simulink model "SetPoint"  (R2023a)
settings: Solver=VariableStepAuto  StartTime=0.0  StopTime=0.2  RelTol=1e-3
values from neighbouring files (symbols this model uses):
  decoupling_active = true    [PMSM.m]
  I_max = 20    [PMSM.m]
  K_Id = R_s/(2*tau_sigma)    (= 675)    [PMSM.m]
  K_Iq = R_s/(2*tau_sigma)    (= 675)    [PMSM.m]
  K_Pd = L_d/(2*tau_sigma)    (= 1.125)    [PMSM.m]
  K_Pq = L_q/(2*tau_sigma)    (= 4.5)    [PMSM.m]
  L_d = 0.00045    [PMSM.m]
  L_q = 0.0018    [PMSM.m]
  motor_type = 1    [PMSM.m]
  p = 4    [PMSM.m]
  Psi_PM = 0.0195    [PMSM.m]
  R_s = 0.27    [PMSM.m]
  Ts = 1 / PWM_frequency    (= 0.0001)    [PMSM.m]
  V_max = V_DC/sqrt(3)    [PMSM.m]
libraries: slpidlib x2
settings Model: PacingRate=0.010000  Creator=brogh  LastModifiedBy=hufnagelde
settings DataIOCC: SaveFormat=StructureWithTime
settings OptimizationCC: ReuseModelBlockBuffer=off
settings DebuggingCC: UnconnectedInputMsg=warning  UnconnectedOutputMsg=warning  UnconnectedLineMsg=warning
settings ModelReferenceCC: EnableRefExpFcnMdlSchedulingChecks=on
settings RTWCC: DLArmComputeVersion=19.05

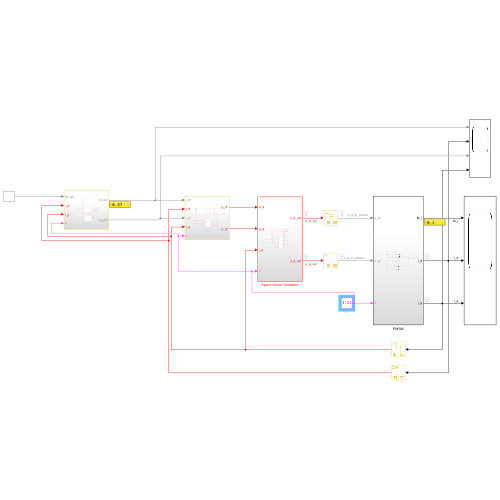
[thumbnail: Simulink's stored preview of the top-level diagram]
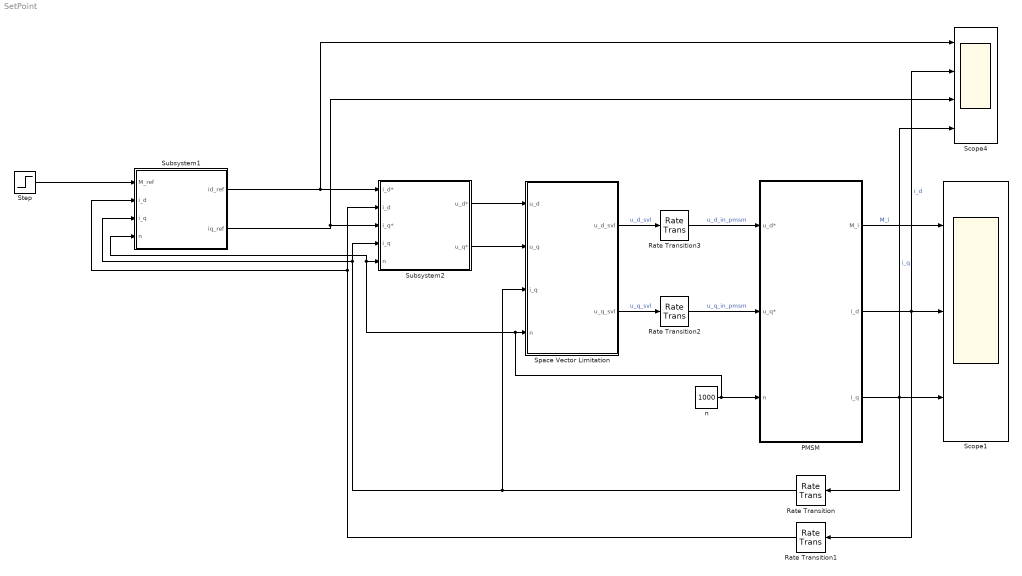
== system SetPoint ==
  PMSM : Subsystem
  Rate Transition : RateTransition  OutPortSampleTime=Ts
  Rate Transition1 : RateTransition  OutPortSampleTime=Ts
  Rate Transition2 : RateTransition  OutPortSampleTime=0
  Rate Transition3 : RateTransition  OutPortSampleTime=0
  Scope1 : Scope  NumInputPorts=3
  Scope4 : Scope  NumInputPorts=4
  Space Vector Limitation : Subsystem
  Step : Step  Time=0.03  After=0.1  SampleTime=0
  Subsystem1 : Subsystem
  Subsystem2 : Subsystem
  n : Constant  Value=1000
  wires:
  PMSM/1(M_i) -> Scope1/1  "M_i"
  PMSM/3(i_q) -> Scope4/4, Scope1/3, Rate Transition/1  "i_q"
  PMSM/2(i_d) -> Scope4/2, Scope1/2, Rate Transition1/1  "i_d"
  Rate Transition/1 -> Subsystem1/3(i_q), Subsystem2/4(i_q), Space Vector Limitation/3(i_q)
  Rate Transition2/1 -> PMSM/2(u_q*)  "u_q_in_pmsm"
  Rate Transition3/1 -> PMSM/1(u_d*)  "u_d_in_pmsm"
  Space Vector Limitation/1(u_d_svl) -> Rate Transition3/1  "u_d_svl"
  Space Vector Limitation/2(u_q_svl) -> Rate Transition2/1  "u_q_svl"
  Subsystem1/1(id_ref) -> Scope4/1, Subsystem2/1(i_d*)
  Subsystem1/2(iq_ref) -> Scope4/3, Subsystem2/3(i_q*)
  Rate Transition1/1 -> Subsystem2/2(i_d), Subsystem1/2(i_d)
  Subsystem2/1(u_d*) -> Space Vector Limitation/1(u_d)
  Subsystem2/2(u_q*) -> Space Vector Limitation/2(u_q)
  Step/1 -> Subsystem1/1(M_ref)
  n/1 -> Subsystem1/4(n), Subsystem2/5(n), Space Vector Limitation/4(n), PMSM/3(n)

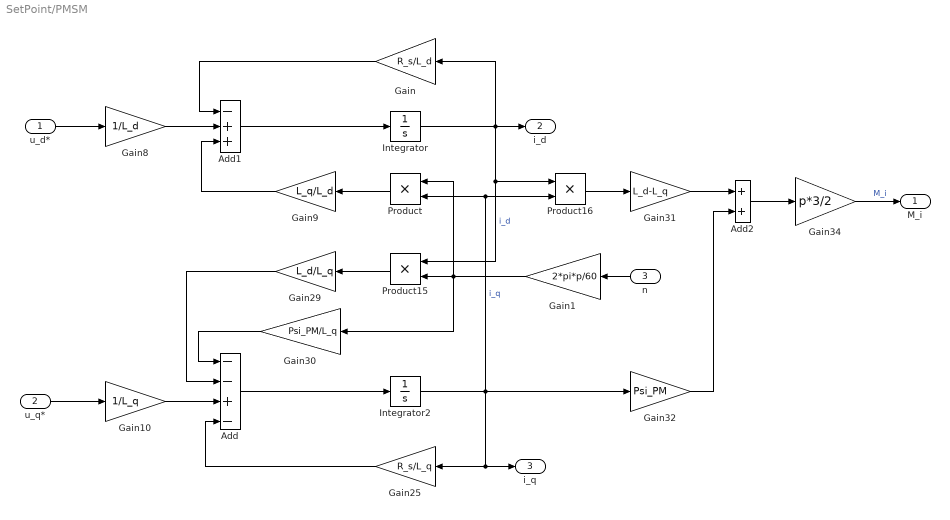
== system SetPoint/PMSM ==
  u_d* : Inport
  u_q* : Inport  Port=2
  n : Inport  Port=3
  Add : Sum  Inputs=--+-
  Add1 : Sum  Inputs=-++
  Add2 : Sum
  Gain : Gain  Gain=R_s/L_d
  Gain1 : Gain  Gain=2*pi*p/60
  Gain10 : Gain  Gain=1/L_q
  Gain25 : Gain  Gain=R_s/L_q
  Gain29 : Gain  Gain=L_d/L_q
  Gain30 : Gain  Gain=Psi_PM/L_q
  Gain31 : Gain  Gain=L_d-L_q
  Gain32 : Gain  Gain=Psi_PM
  Gain34 : Gain  Gain=p*3/2
  Gain8 : Gain  Gain=1/L_d
  Gain9 : Gain  Gain=L_q/L_d
  Integrator : Integrator
  Integrator2 : Integrator
  Product : Product
  Product15 : Product
  Product16 : Product
  M_i : Outport
  i_d : Outport  Port=2
  i_q : Outport  Port=3
  wires:
  n/1 -> Gain1/1
  Add2/1 -> Gain34/1
  u_d*/1 -> Gain8/1
  Integrator/1 -> i_d/1, Product16/1, Product15/1, Gain/1  "i_d"
  Gain34/1 -> M_i/1  "M_i"
  Gain25/1 -> Add/4
  Product15/1 -> Gain29/1
  Add1/1 -> Integrator/1
  Add/1 -> Integrator2/1
  Gain9/1 -> Add1/3
  Gain8/1 -> Add1/2
  Gain10/1 -> Add/3
  Gain32/1 -> Add2/2
  Gain/1 -> Add1/1
  u_q*/1 -> Gain10/1
  Product/1 -> Gain9/1
  Gain29/1 -> Add/2
  Gain31/1 -> Add2/1
  Product16/1 -> Gain31/1
  Integrator2/1 -> i_q/1, Gain25/1, Gain32/1, Product/2, Product16/2  "i_q"
  Gain30/1 -> Add/1
  Gain1/1 -> Gain30/1, Product/1, Product15/2

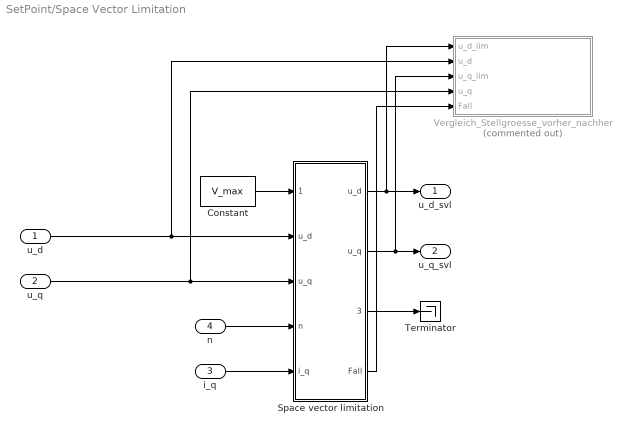
== system SetPoint/Space Vector Limitation ==
  u_d : Inport
  u_q : Inport  Port=2
  i_q : Inport  Port=3
  n : Inport  Port=4
  Constant : Constant  Value=V_max
  Space vector limitation : MATLAB Function  TreatAsAtomicUnit=on
  Terminator : Terminator
  Vergleich_Stellgroesse_vorher_nachher : Subsystem  Commented=on
  u_d_svl : Outport
  u_q_svl : Outport  Port=2
  wires:
  u_d/1 -> Space vector limitation/2("u_d "), Vergleich_Stellgroesse_vorher_nachher/2(u_d)
  u_q/1 -> Vergleich_Stellgroesse_vorher_nachher/4(u_q), Space vector limitation/3("u_q ")
  n/1 -> Space vector limitation/4(n)
  Space vector limitation/1(u_d) -> u_d_svl/1, Vergleich_Stellgroesse_vorher_nachher/1(u_d_lim)
  Constant/1 -> Space vector limitation/1(U_max)
  Space vector limitation/3(limit_on) -> Terminator/1
  i_q/1 -> Space vector limitation/5(i_q)
  Space vector limitation/2(u_q) -> u_q_svl/1, Vergleich_Stellgroesse_vorher_nachher/3(u_q_lim)
  Space vector limitation/4(Fall) -> Vergleich_Stellgroesse_vorher_nachher/5(Fall)

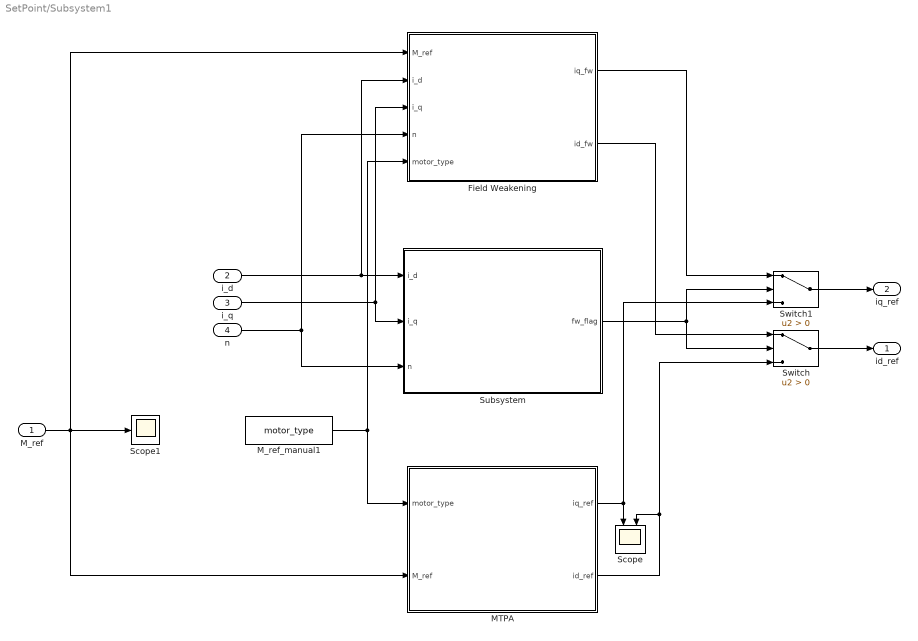
== system SetPoint/Subsystem1 ==
  M_ref : Inport
  i_d : Inport  Port=2
  i_q : Inport  Port=3
  n : Inport  Port=4
  Field Weakening : Subsystem
  MTPA : Subsystem
  M_ref_manual1 : Constant  Value=motor_type  OutDataTypeStr=single
  Scope : Scope  NumInputPorts=2
  Scope1 : Scope
  Subsystem : Subsystem
  Switch : Switch  Criteria=u2 > Threshold  SaturateOnIntegerOverflow=off  InputSameDT=off
  Switch1 : Switch  Criteria=u2 > Threshold  SaturateOnIntegerOverflow=off  InputSameDT=off
  id_ref : Outport
  iq_ref : Outport  Port=2
  wires:
  MTPA/1(iq_ref) -> Switch1/3, Scope/1
  MTPA/2(id_ref) -> Switch/3, Scope/2
  M_ref/1 -> MTPA/2(M_ref), Scope1/1, Field Weakening/1(M_ref)
  M_ref_manual1/1 -> MTPA/1(motor_type), Field Weakening/5(motor_type)
  i_d/1 -> Subsystem/1(i_d), Field Weakening/2(i_d)
  i_q/1 -> Subsystem/2(i_q), Field Weakening/3(i_q)
  n/1 -> Subsystem/3(n), Field Weakening/4(n)
  Subsystem/1(fw_flag) -> Switch/2, Switch1/2
  Field Weakening/1(iq_fw) -> Switch1/1
  Field Weakening/2(id_fw) -> Switch/1
  Switch1/1 -> iq_ref/1
  Switch/1 -> id_ref/1

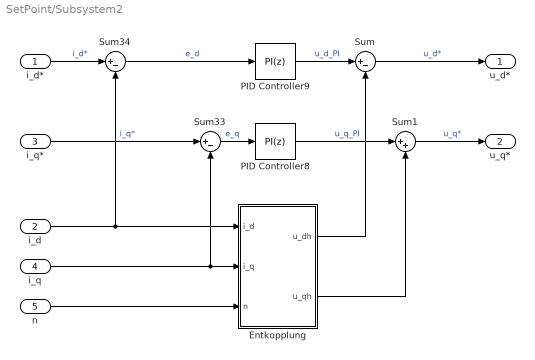
== system SetPoint/Subsystem2 ==
  i_d* : Inport
  i_d : Inport  Port=2
  i_q* : Inport  Port=3
  i_q : Inport  Port=4
  n : Inport  Port=5
  Entkopplung : Subsystem
  PID Controller8 : slpidlib/PID Controller  Controller=PI  Form=Parallel  TimeDomain=Discrete-time  UseExternalTs=off  SampleTime=Ts  IntegratorMethod=Forward Euler  FilterMethod=Forward Euler  ControllerParametersSource=internal  P=K_Pq  I=K_Iq  UseKiTs=off  D=0  N=100  UseFilter=on  TunerSelectOption=Transfer Function Based (PID Tuner App)  InitialConditionSource=internal  InitialConditionForIntegrator=0  InitialConditionForFilter=0  DifferentiatorICPrevScaledInput=0  ExternalReset=none  TrackingMode=off  Kt=1  LimitOutput=on  SatLimitsSource=internal  UpperSaturationLimit=V_max  LowerSaturationLimit=-V_max  LinearizeAsGain=on  AntiWindupMode=clamping  Kb=1  LimitIntegrator=off  UpperIntegratorSaturationLimit=inf  LowerIntegratorSaturationLimit=-inf  POutMin=[]  POutMax=[]  IOutMin=[]  IOutMax=[]  DOutMin=[]  DOutMax=[]  NOutMin=[]  NOutMax=[]  SumOutMin=[]  SumOutMax=[]  SaturationOutMin=[]  SaturationOutMax=[]  PParamMin=[]  PParamMax=[]  IParamMin=[]  IParamMax=[]  DParamMin=[]  DParamMax=[]  NParamMin=[]  NParamMax=[]  KbParamMin=[]  KbParamMax=[]  KtParamMin=[]  KtParamMax=[]  KbOutMin=[]  KbOutMax=[]  KtOutMin=[]  KtOutMax=[]  IntegratorOutMin=[]  IntegratorOutMax=[]  FilterOutMin=[]  FilterOutMax=[]  SumI1OutMin=[]  SumI1OutMax=[]  SumI2OutMin=[]  SumI2OutMax=[]  SumI3OutMin=[]  SumI3OutMax=[]  SumI4OutMin=[]  SumI4OutMax=[]  SumDOutMin=[]  SumDOutMax=[]  DifferentiatorOutMin=[]  DifferentiatorOutMax=[]  FilterDiffOutCoefMin=[]  FilterDiffOutCoefMax=[]  ReciprocalOutMin=[]  ReciprocalOutMax=[]  SumDenOutMin=[]  SumDenOutMax=[]  SumNumOutMin=[]  SumNumOutMax=[]  DivideOutMin=[]  DivideOutMax=[]  UdiffTsProdOutMin=[]  UdiffTsProdOutMax=[]  NTsProdOutMin=[]  NTsProdOutMax=[]  UintegralTsProdOutMin=[]  UintegralTsProdOutMax=[]  UngainTsProdOutMin=[]  UngainTsProdOutMax=[]  ClampingZeroOutDataTypeStr=Inherit: Inherit via back propagation  ClampingZeroOutMin=[]  ClampingZeroOutMax=[]  FilterDenConstantOutDataTypeStr=Inherit: Inherit via back propagation  FilterDenConstantOutMin=[]  FilterDenConstantOutMax=[]  PCopyOutDataTypeStr=Inherit: Inherit via back propagation  PCopyOutMin=[]  PCopyOutMax=[]  NCopyOutDataTypeStr=Inherit: Inherit via back propagation  NCopyOutMin=[]  NCopyOutMax=[]  IntegratorContinuousStateAttributes=''  IntegratorStateMustResolveToSignalObject=off  IntegratorRTWStateStorageClass=Auto  FilterContinuousStateAttributes=''  FilterStateMustResolveToSignalObject=off  FilterRTWStateStorageClass=Auto  ParallelPVariant=InternalParameters  IdealPVariant=Disabled  IVariant=InternalParameters  DVariant=Disabled  IntegratorVariant=Discrete  SatVariant=Enabled  AWVariant=DiscClampingParallel  PCopyVariant=Disabled  TRVariant=Disabled  FdbkBlocksVariant=Forward  IdealPFdbkVariant=Disabled  SatFdbkVariant=Disabled  DerivativeFilterVariant=Disabled  NVariant=Disabled  NCopyVariant=Disabled_SignalSpec  FilterICVariant=Disabled  IntegratorICVariant=InternalICs  ExternalResetVariant=Disabled  TRSumVariant=Passthrough  SumFdbkVariant=Disabled  SumVariant=Sum_PI  TsampFilterVariant=InternalTs  TsampNgainVariant=Passthrough  TsampIntegralVariant=Disabled_SignalSpec  ExternalSaturationOutDataTypeStr=Inherit: Same as second input
  PID Controller9 : slpidlib/PID Controller  Controller=PI  Form=Parallel  TimeDomain=Discrete-time  UseExternalTs=off  SampleTime=Ts  IntegratorMethod=Forward Euler  FilterMethod=Forward Euler  ControllerParametersSource=internal  P=K_Pd  I=K_Id  UseKiTs=off  D=0  N=100  UseFilter=on  TunerSelectOption=Transfer Function Based (PID Tuner App)  InitialConditionSource=internal  InitialConditionForIntegrator=0  InitialConditionForFilter=0  DifferentiatorICPrevScaledInput=0  ExternalReset=none  TrackingMode=off  Kt=1  LimitOutput=on  SatLimitsSource=internal  UpperSaturationLimit=V_max  LowerSaturationLimit=-V_max  LinearizeAsGain=on  AntiWindupMode=clamping  Kb=1  LimitIntegrator=off  UpperIntegratorSaturationLimit=inf  LowerIntegratorSaturationLimit=-inf  POutMin=[]  POutMax=[]  IOutMin=[]  IOutMax=[]  DOutMin=[]  DOutMax=[]  NOutMin=[]  NOutMax=[]  SumOutMin=[]  SumOutMax=[]  SaturationOutMin=[]  SaturationOutMax=[]  PParamMin=[]  PParamMax=[]  IParamMin=[]  IParamMax=[]  DParamMin=[]  DParamMax=[]  NParamMin=[]  NParamMax=[]  KbParamMin=[]  KbParamMax=[]  KtParamMin=[]  KtParamMax=[]  KbOutMin=[]  KbOutMax=[]  KtOutMin=[]  KtOutMax=[]  IntegratorOutMin=[]  IntegratorOutMax=[]  FilterOutMin=[]  FilterOutMax=[]  SumI1OutMin=[]  SumI1OutMax=[]  SumI2OutMin=[]  SumI2OutMax=[]  SumI3OutMin=[]  SumI3OutMax=[]  SumI4OutMin=[]  SumI4OutMax=[]  SumDOutMin=[]  SumDOutMax=[]  DifferentiatorOutMin=[]  DifferentiatorOutMax=[]  FilterDiffOutCoefMin=[]  FilterDiffOutCoefMax=[]  ReciprocalOutMin=[]  ReciprocalOutMax=[]  SumDenOutMin=[]  SumDenOutMax=[]  SumNumOutMin=[]  SumNumOutMax=[]  DivideOutMin=[]  DivideOutMax=[]  UdiffTsProdOutMin=[]  UdiffTsProdOutMax=[]  NTsProdOutMin=[]  NTsProdOutMax=[]  UintegralTsProdOutMin=[]  UintegralTsProdOutMax=[]  UngainTsProdOutMin=[]  UngainTsProdOutMax=[]  ClampingZeroOutDataTypeStr=Inherit: Inherit via back propagation  ClampingZeroOutMin=[]  ClampingZeroOutMax=[]  FilterDenConstantOutDataTypeStr=Inherit: Inherit via back propagation  FilterDenConstantOutMin=[]  FilterDenConstantOutMax=[]  PCopyOutDataTypeStr=Inherit: Inherit via back propagation  PCopyOutMin=[]  PCopyOutMax=[]  NCopyOutDataTypeStr=Inherit: Inherit via back propagation  NCopyOutMin=[]  NCopyOutMax=[]  IntegratorContinuousStateAttributes=''  IntegratorStateMustResolveToSignalObject=off  IntegratorRTWStateStorageClass=Auto  FilterContinuousStateAttributes=''  FilterStateMustResolveToSignalObject=off  FilterRTWStateStorageClass=Auto  ParallelPVariant=InternalParameters  IdealPVariant=Disabled  IVariant=InternalParameters  DVariant=Disabled  IntegratorVariant=Discrete  SatVariant=Enabled  AWVariant=DiscClampingParallel  PCopyVariant=Disabled  TRVariant=Disabled  FdbkBlocksVariant=Forward  IdealPFdbkVariant=Disabled  SatFdbkVariant=Disabled  DerivativeFilterVariant=Disabled  NVariant=Disabled  NCopyVariant=Disabled_SignalSpec  FilterICVariant=Disabled  IntegratorICVariant=InternalICs  ExternalResetVariant=Disabled  TRSumVariant=Passthrough  SumFdbkVariant=Disabled  SumVariant=Sum_PI  TsampFilterVariant=InternalTs  TsampNgainVariant=Passthrough  TsampIntegralVariant=Disabled_SignalSpec  ExternalSaturationOutDataTypeStr=Inherit: Same as second input
  Sum : Sum  Inputs=|+-
  Sum1 : Sum  Inputs=|++
  Sum33 : Sum  Inputs=|+-
  Sum34 : Sum  Inputs=|+-
  u_d* : Outport
  u_q* : Outport  Port=2
  wires:
  Entkopplung/2(u_qh) -> Sum1/2
  Sum34/1 -> PID Controller9/1  "e_d"
  i_d/1 -> Sum34/2, Entkopplung/1(i_d)
  i_d*/1 -> Sum34/1  "i_d*"
  i_q/1 -> Sum33/2, Entkopplung/2(i_q)
  PID Controller8/1 -> Sum1/1  "u_q_PI"
  i_q*/1 -> Sum33/1  "i_q*"
  n/1 -> Entkopplung/3(n)
  Entkopplung/1(u_dh) -> Sum/2
  Sum/1 -> u_d*/1  "u_d*"
  PID Controller9/1 -> Sum/1  "u_d_PI"
  Sum1/1 -> u_q*/1  "u_q*"
  Sum33/1 -> PID Controller8/1  "e_q"

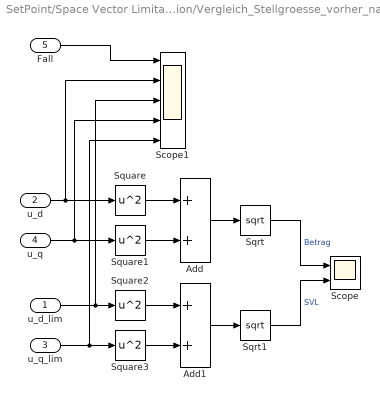
== system SetPoint/Space Vector Limitation/Vergleich_Stellgroesse_vorher_nachher ==
  u_d_lim : Inport
  u_d : Inport  Port=2
  u_q_lim : Inport  Port=3
  u_q : Inport  Port=4
  Fall : Inport  Port=5
  Add : Sum
  Add1 : Sum
  Scope : Scope  NumInputPorts=2
  Scope1 : Scope  NumInputPorts=5
  Sqrt : Sqrt
  Sqrt1 : Sqrt
  Square{,1..3} (4 alike) : Math  Operator=square
  wires:
  Square3/1 -> Add1/2
  Add/1 -> Sqrt/1
  Sqrt1/1 -> Scope/2  "SVL"
  Square2/1 -> Add1/1
  Square/1 -> Add/1
  Add1/1 -> Sqrt1/1
  Square1/1 -> Add/2
  Sqrt/1 -> Scope/1  "Betrag"
  u_d_lim/1 -> Scope1/3, Square2/1
  u_d/1 -> Scope1/2, Square/1
  u_q/1 -> Scope1/4, Square1/1
  u_q_lim/1 -> Scope1/5, Square3/1
  Fall/1 -> Scope1/1

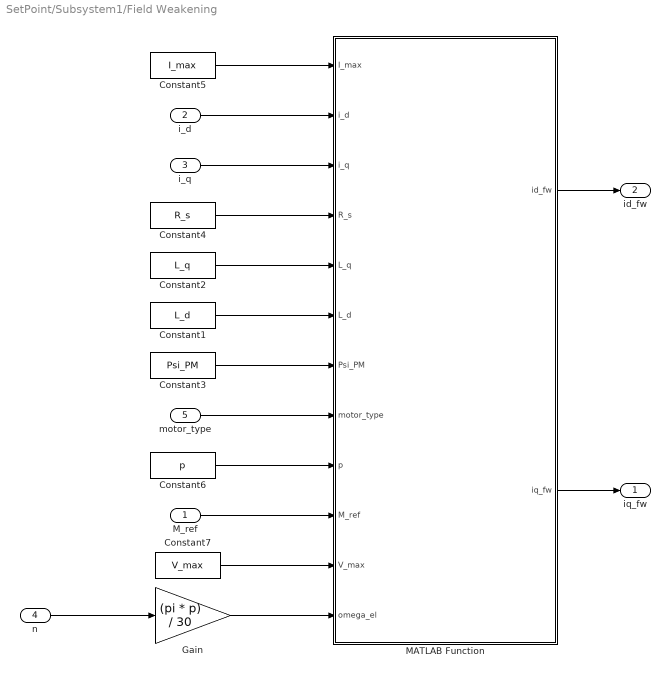
== system SetPoint/Subsystem1/Field Weakening ==
  M_ref : Inport
  i_d : Inport  Port=2
  i_q : Inport  Port=3
  n : Inport  Port=4
  motor_type : Inport  Port=5
  Constant1 : Constant  Value=L_d
  Constant2 : Constant  Value=L_q
  Constant3 : Constant  Value=Psi_PM
  Constant4 : Constant  Value=R_s
  Constant5 : Constant  Value=I_max
  Constant6 : Constant  Value=p
  Constant7 : Constant  Value=V_max
  Gain : Gain  Gain=(pi * p) / 30
  MATLAB Function : MATLAB Function  TreatAsAtomicUnit=on
  iq_fw : Outport
  id_fw : Outport  Port=2
  wires:
  Constant5/1 -> MATLAB Function/1(I_max)
  Constant4/1 -> MATLAB Function/4(R_s)
  Constant2/1 -> MATLAB Function/5(L_q)
  Constant1/1 -> MATLAB Function/6(L_d)
  Constant3/1 -> MATLAB Function/7(Psi_PM)
  MATLAB Function/2(iq_fw) -> iq_fw/1
  MATLAB Function/1(id_fw) -> id_fw/1
  motor_type/1 -> MATLAB Function/8(motor_type)
  M_ref/1 -> MATLAB Function/10(M_ref)
  Constant6/1 -> MATLAB Function/9(p)
  i_d/1 -> MATLAB Function/2(i_d)
  i_q/1 -> MATLAB Function/3(i_q)
  Constant7/1 -> MATLAB Function/11(V_max)
  n/1 -> Gain/1
  Gain/1 -> MATLAB Function/12(omega_el)

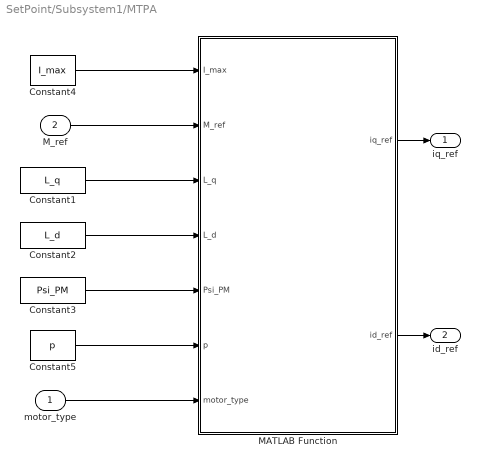
== system SetPoint/Subsystem1/MTPA ==
  motor_type : Inport
  M_ref : Inport  Port=2
  Constant1 : Constant  Value=L_q
  Constant2 : Constant  Value=L_d
  Constant3 : Constant  Value=Psi_PM
  Constant4 : Constant  Value=I_max
  Constant5 : Constant  Value=p
  MATLAB Function : MATLAB Function  TreatAsAtomicUnit=on
  iq_ref : Outport
  id_ref : Outport  Port=2
  wires:
  Constant4/1 -> MATLAB Function/1(I_max)
  Constant1/1 -> MATLAB Function/3(L_q)
  Constant2/1 -> MATLAB Function/4(L_d)
  Constant3/1 -> MATLAB Function/5(Psi_PM)
  MATLAB Function/2(id_ref) -> id_ref/1
  MATLAB Function/1(iq_ref) -> iq_ref/1
  motor_type/1 -> MATLAB Function/7(motor_type)
  Constant5/1 -> MATLAB Function/6(p)
  M_ref/1 -> MATLAB Function/2(M_ref)

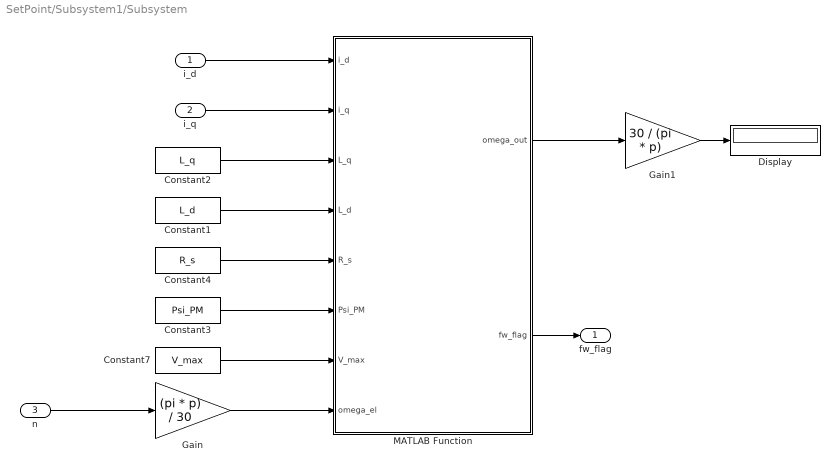
== system SetPoint/Subsystem1/Subsystem ==
  i_d : Inport
  i_q : Inport  Port=2
  n : Inport  Port=3
  Constant1 : Constant  Value=L_d
  Constant2 : Constant  Value=L_q
  Constant3 : Constant  Value=Psi_PM
  Constant4 : Constant  Value=R_s
  Constant7 : Constant  Value=V_max
  Display : Display
  Gain : Gain  Gain=(pi * p) / 30
  Gain1 : Gain  Gain=30 / (pi * p)
  MATLAB Function : MATLAB Function  TreatAsAtomicUnit=on
  fw_flag : Outport
  wires:
  Constant3/1 -> MATLAB Function/6(Psi_PM)
  i_d/1 -> MATLAB Function/1(i_d)
  Constant7/1 -> MATLAB Function/7(V_max)
  i_q/1 -> MATLAB Function/2(i_q)
  n/1 -> Gain/1
  Gain/1 -> MATLAB Function/8(omega_el)
  Constant4/1 -> MATLAB Function/5(R_s)
  Constant1/1 -> MATLAB Function/4(L_d)
  Constant2/1 -> MATLAB Function/3(L_q)
  MATLAB Function/2(fw_flag) -> fw_flag/1
  MATLAB Function/1(omega_out) -> Gain1/1
  Gain1/1 -> Display/1

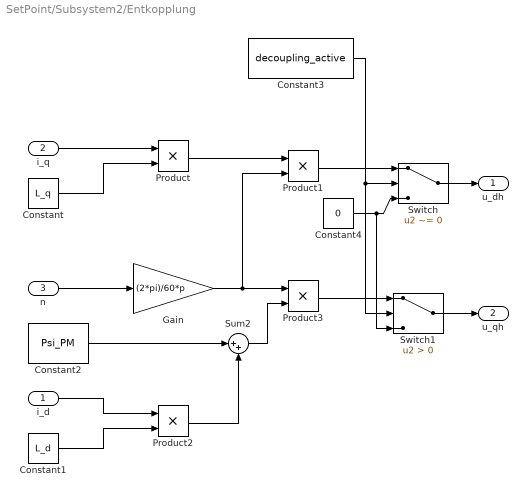
== system SetPoint/Subsystem2/Entkopplung ==
  i_d : Inport
  i_q : Inport  Port=2
  n : Inport  Port=3
  Constant : Constant  Value=L_q
  Constant1 : Constant  Value=L_d
  Constant2 : Constant  Value=Psi_PM
  Constant3 : Constant  Value=decoupling_active
  Constant4 : Constant  Value=0
  Gain : Gain  Gain=(2*pi)/60*p
  Product{,1..3} (4 alike) : Product
  Sum2 : Sum  Inputs=|++
  Switch : Switch  Criteria=u2 ~= 0  SaturateOnIntegerOverflow=off  InputSameDT=off
  Switch1 : Switch  Criteria=u2 > Threshold  SaturateOnIntegerOverflow=off  InputSameDT=off
  u_dh : Outport
  u_qh : Outport  Port=2
  wires:
  Gain/1 -> Product3/1, Product1/2
  Sum2/1 -> Product3/2
  Constant/1 -> Product/2
  n/1 -> Gain/1
  Product2/1 -> Sum2/2
  Constant2/1 -> Sum2/1
  Constant1/1 -> Product2/2
  Product1/1 -> Switch/1
  Product/1 -> Product1/1
  i_d/1 -> Product2/1
  i_q/1 -> Product/1
  Product3/1 -> Switch1/1
  Constant3/1 -> Switch/2, Switch1/2
  Constant4/1 -> Switch1/3, Switch/3
  Switch/1 -> u_dh/1
  Switch1/1 -> u_qh/1

== matlab function SetPoint/Subsystem1/Subsystem/MATLAB Function ==
  settings: updateMethod=DISCRETE
  data: i_d input; i_q input; omega_out output; L_q input; L_d input; R_s input; Psi_PM input; fw_flag output; V_max input; omega_el input
function [omega_out, fw_flag]= Omega_Cut_Calculation(i_d, i_q, L_q, L_d, R_s, Psi_PM, V_max, omega_el)


persistent omega_cut
if isempty(omega_cut)
    omega_cut = 0;
end
V_max = V_max * 0.95;
a = L_q^2 * i_q^2 + Psi_PM^2 + L_d * i_d * (2 * Psi_PM + L_d * i_d);
b = 2 * R_s * i_q * (i_d * (L_d - L_q) + Psi_PM);
c = R_s^2 * (i_d^2 + i_q^2) - V_max^2;

omega_out = (-b + sqrt(b^2 - 4 * a * c)) / (2 * a);

if (omega_cut == 0)
    omega_cut = omega_out;
end

if ( abs(omega_el) < omega_cut)
    omega_cut = omega_out;
    fw_flag = false;
else
    if(omega_el < 0)
        omega_out = -omega_cut;
    else
        omega_out = omega_cut;
    end 
    fw_flag = true;
end



end

== matlab function SetPoint/Space Vector Limitation/Space vector limitation ==
  data: U_max input; u_d input; u_d output; u_q input; u_q output; n input; i_q input; limit_on output; Fall output
function [u_d, u_q, limit_on, Fall] = fcn(U_max, u_d, u_q, n, i_q)

U_abs = sqrt(u_d^2 + u_q^2); % tatsächlicher Betrag des Spannungsraumzeigers

% Ist eine Begrenzung notwendig?
if ( U_abs > U_max )
    limit_on = boolean(1);
    
    % Motor- oder Generatorbetrieb?
    if ((sign(n))==(sign(i_q))) % Motorbetrieb

        if (abs(u_d) > (0.95*U_max))
            u_d_lim = sign(u_d) * 0.95 * U_max;
            u_q_lim = sign(u_q) * sqrt(U_max^2 - u_d_lim^2);
            Fall=1;
        else
            u_d_lim = u_d;
            u_q_lim = sign(u_q) * sqrt(U_max^2 - u_d_lim^2);
            Fall=2;
        end
    

    else % Generatorbetrieb
        
        if ((abs(u_q)) > (0.95*U_max))
            u_q_lim = sign(u_q) * 0.95 * U_max;
            u_d_lim = sign(u_d) * sqrt(U_max^2 - u_q_lim^2);
            Fall=3;
        else
            u_q_lim = u_q;
            u_d_lim = sign(u_d) * sqrt(U_max^2 - u_q_lim^2);
            Fall=4;
        end

    end    

else % keine Begrenzung nötig
    u_d_lim = u_d;
    u_q_lim = u_q;
    limit_on = boolean(0);
    Fall=5;
end

u_d = u_d_lim;
u_q = u_q_lim;

end

== matlab function SetPoint/Subsystem1/MTPA/MATLAB Function ==
  data: I_max input; M_ref input; iq_ref output; L_q input; L_d input; Psi_PM input; p input; id_ref output; motor_type input
function [iq_ref, id_ref]= MTPA(I_max, M_ref, L_q, L_d, Psi_PM, p, motor_type)
if (M_ref ~= 0)
    
    if(motor_type==0)
        iq_ref = M_ref/(1.5*p*Psi_PM);
        iq_ref = min(I_max, max(-I_max, iq_ref));
        id_ref = 0;
    elseif(motor_type==1)
        d = 2*M_ref*Psi_PM/(3*(L_d-L_q)^2*p);
        e = -(2*M_ref)^2/(9*(L_d-L_q)^2*p^2);
        iq_polynom = [1 0 0 d e]; % Schröder, Regelung von Antriebssystemen, S. 1110
        iq_ref = real(min(roots(iq_polynom)));
        iq_ref = min(I_max, max(-I_max, iq_ref));
        if (L_q > L_d)
            id_temp = (-Psi_PM / (2*(L_d - L_q))) - sqrt((Psi_PM^2 / (4*(L_d - L_q)^2))+iq_ref^2 );
            id_ref = max(id_temp, -sqrt(I_max^2 - iq_ref^2));
        else
            id_temp = (-Psi_PM / (2*(L_d - L_q))) + sqrt((Psi_PM^2 / (4*(L_d - L_q)^2))+iq_ref^2 );
            id_ref = min(id_temp, sqrt(I_max^2 - iq_ref^2));
        end
    else
        id_ref = 0;
        iq_ref = 0;
    end
else
    id_ref = 0;
    iq_ref = 0;
end

== matlab function SetPoint/Subsystem1/Field Weakening/MATLAB Function ==
  data: I_max input; id_fw output; i_d input; i_q input; R_s input; L_q input; L_d input; Psi_PM input; iq_fw output; motor_type input; p input; M_ref input; V_max input; omega_el input
function [id_fw, iq_fw]= field_weakening(I_max, i_d, i_q, R_s, L_q, L_d, Psi_PM, motor_type, p, M_ref, V_max, omega_el)


%Maximum voltage vector
I1 = sqrt(i_q^2 + i_d^2);
V_FE_max = (V_max - R_s*I1) * 0.95;

if(M_ref ~=0)
        %Calcultation of Id_ref
            if(motor_type == 0)
                iq_fw = M_ref/(1.5*p*Psi_PM);
                iq_fw = min(I_max, max(-I_max, iq_fw));
                id_fw = (-Psi_PM / L_d) + (1 / L_d) * sqrt((V_FE_max / omega_el)^2 - (L_q * iq_fw)^2);
                id_fw = max(id_fw, -I_max);
            elseif(motor_type == 1)
                c =  (Psi_PM^2 * L_q^2 - (L_d - L_q)^2 * (V_FE_max / omega_el)^2) / (L_q^2 * (L_d - L_q)^2);
                d = (-4 * M_ref * L_d * L_q * Psi_PM) / (3 * L_q^2 * p * (L_d - L_q)^2);
                e = (4 * (M_ref * L_d)^2) / (9 * L_q^2 * p^2 * (L_d - L_q)^2);
                iq_polynom = [1 0 c d e]; % Schröder, Regelung von Antriebssystemen, S. 1110
                if (omega_el < 0)
                    iq_fw = min(real(roots(iq_polynom)));
                else
                    iq_fw = max(real(roots(iq_polynom)));
                end
                
                if(iq_fw <0)           
                    iq_fw = max(iq_fw, -I_max);
                else          
                    iq_fw = min(iq_fw, I_max);
                end     
                id_fw = (-Psi_PM / L_d) + (1 / L_d) * sqrt((V_FE_max / omega_el)^2 - (L_q * iq_fw)^2);
            else
                id_fw = 0.0;
                iq_fw = 0.0;
            end
            id_fw = max(id_fw, -sqrt(I_max^2 - iq_fw^2));
            if id_fw > 0
                id_fw = 0.0;
            end

else
    id_fw = 0.0;
    iq_fw = 0.0;
end
